simulink model "state_space_model_v0021"  (R2022b)
settings: Solver=VariableStepAuto  StartTime=0.0  StopTime=100  RelTol=1e-3
undefined symbols (not defined in the file): A_num, b_num, c, DiscIntNeverNeededParam, F_new, G, init_cond, Ts
libraries: simulink x1
settings Model: Creator=ninj2  LastModifiedBy=ninj2

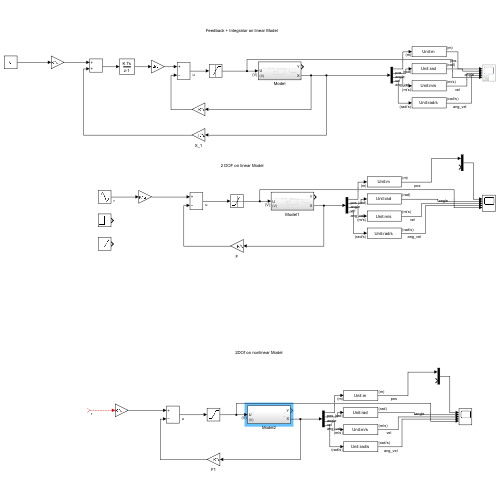
[thumbnail: Simulink's stored preview of the top-level diagram]
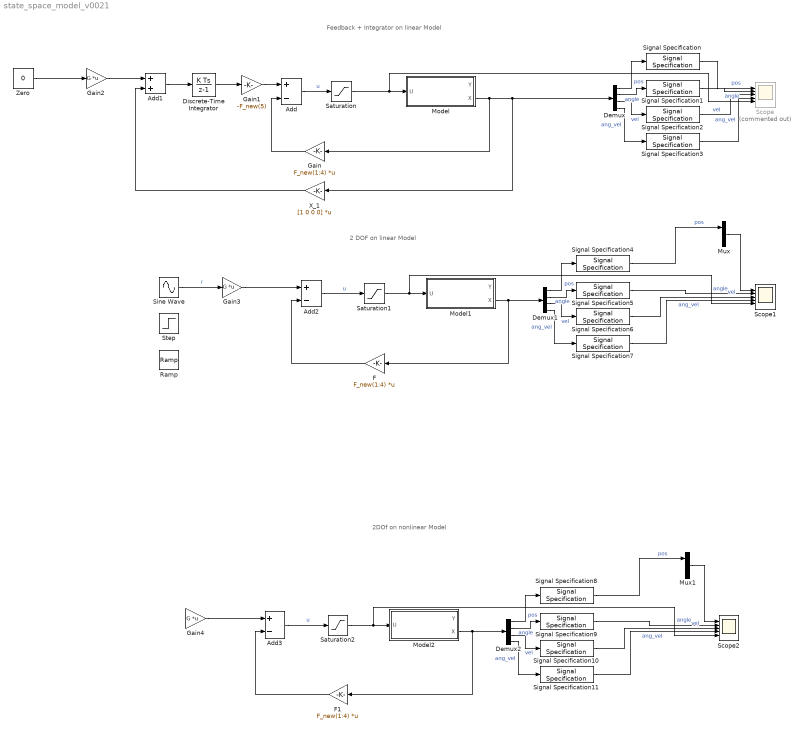
== system state_space_model_v0021 ==
  note: 2DOf on nonlinear Model
  note: 2 DOF on linear Model
  note: Feedback + Integrator on linear Model
  Add : Sum  Inputs=+-
  Add1 : Sum
  Add2 : Sum  Inputs=+-
  Add3 : Sum  Inputs=+-
  Demux : Demux
  Demux1 : Demux
  Demux2 : Demux
  Discrete-Time Integrator : DiscreteIntegrator  SampleTime=-1  ICPrevOutput=DiscIntNeverNeededParam  ICPrevScaledInput=DiscIntNeverNeededParam
  F : Gain  Gain=F_new(1:4)  Multiplication=Matrix(K*u)
  F1 : Gain  Gain=F_new(1:4)  Multiplication=Matrix(K*u)
  Gain : Gain  Gain=F_new(1:4)  Multiplication=Matrix(K*u)
  Gain1 : Gain  Gain=-F_new(5)
  Gain2 : Gain  Gain=G  Multiplication=Matrix(K*u)
  Gain3 : Gain  Gain=G  Multiplication=Matrix(K*u)
  Gain4 : Gain  Gain=G  Multiplication=Matrix(K*u)
  Model : Subsystem
  Model1 : Subsystem
  Model2 : Subsystem
  Mux : Mux  Inputs=2
  Mux1 : Mux  Inputs=2
  Ramp : simulink/Sources/Ramp  slope=0.01  start=0  InitialOutput=0
  Saturation : Saturate  UpperLimit=9  LowerLimit=-9
  Saturation1 : Saturate  UpperLimit=9  LowerLimit=-9
  Saturation2 : Saturate  UpperLimit=9  LowerLimit=-9
  Scope : Scope  Commented=on  NumInputPorts=5
  Scope1 : Scope  NumInputPorts=5
  Scope2 : Scope  NumInputPorts=5
  Signal Specification : SignalSpecification  Unit=m
  Signal Specification1 : SignalSpecification  Unit=rad
  Signal Specification10 : SignalSpecification  Unit=m/s
  Signal Specification11 : SignalSpecification  Unit=rad/s
  Signal Specification2 : SignalSpecification  Unit=m/s
  Signal Specification3 : SignalSpecification  Unit=rad/s
  Signal Specification4 : SignalSpecification  Unit=m
  Signal Specification5 : SignalSpecification  Unit=rad
  Signal Specification6 : SignalSpecification  Unit=m/s
  Signal Specification7 : SignalSpecification  Unit=rad/s
  Signal Specification8 : SignalSpecification  Unit=m
  Signal Specification9 : SignalSpecification  Unit=rad
  Sine Wave : Sin  Amplitude=0.05  Frequency=0.3  SampleTime=0
  Step : Step  After=0.05  SampleTime=0
  X_1 : Gain  Gain=[1 0 0 0]  Multiplication=Matrix(K*u)
  Zero : Constant  Value=0  OutDataTypeStr=Inherit: Inherit via back propagation
  wires:
  Add/1 -> Saturation/1  "u"
  Model/2(X) -> Gain/1, X_1/1, Demux/1
  Gain/1 -> Add/2
  Zero/1 -> Gain2/1
  Add1/1 -> Discrete-Time Integrator/1
  Discrete-Time Integrator/1 -> Gain1/1
  X_1/1 -> Add1/2
  Gain1/1 -> Add/1
  Demux/1 -> Signal Specification/1  "pos"
  Demux/2 -> Signal Specification1/1  "angle"
  Demux/3 -> Signal Specification2/1  "vel"
  Demux/4 -> Signal Specification3/1  "ang_vel"
  Signal Specification/1 -> Scope/1  "pos"
  Signal Specification1/1 -> Scope/2  "angle"
  Signal Specification2/1 -> Scope/3  "vel"
  Signal Specification3/1 -> Scope/4  "ang_vel"
  Saturation/1 -> Scope/5, Model/1(U)
  Saturation1/1 -> Scope1/5, Model1/1(U)
  Add2/1 -> Saturation1/1  "u"
  Demux1/1 -> Signal Specification4/1  "pos"
  Signal Specification7/1 -> Scope1/4  "ang_vel"
  Signal Specification6/1 -> Scope1/3  "vel"
  F/1 -> Add2/2
  Demux1/3 -> Signal Specification6/1  "vel"
  Signal Specification4/1 -> Mux/1  "pos"
  Demux1/4 -> Signal Specification7/1  "ang_vel"
  Signal Specification5/1 -> Scope1/2  "angle"
  Model1/2(X) -> F/1, Demux1/1
  Demux1/2 -> Signal Specification5/1  "angle"
  Gain3/1 -> Add2/1
  Mux/1 -> Scope1/1
  Gain2/1 -> Add1/1
  Sine Wave/1 -> Gain3/1  "r"
  Demux2/3 -> Signal Specification10/1  "vel"
  Signal Specification9/1 -> Scope2/2  "angle"
  Mux1/1 -> Scope2/1
  Demux2/4 -> Signal Specification11/1  "ang_vel"
  Gain4/1 -> Add3/1
  Signal Specification11/1 -> Scope2/4  "ang_vel"
  Demux2/2 -> Signal Specification9/1  "angle"
  Model2/2(X) -> F1/1, Demux2/1
  ? -> Gain4/1  "r"
  Saturation2/1 -> Scope2/5, Model2/1(U)
  Signal Specification8/1 -> Mux1/1  "pos"
  Demux2/1 -> Signal Specification8/1  "pos"
  F1/1 -> Add3/2
  Signal Specification10/1 -> Scope2/3  "vel"
  Add3/1 -> Saturation2/1  "u"

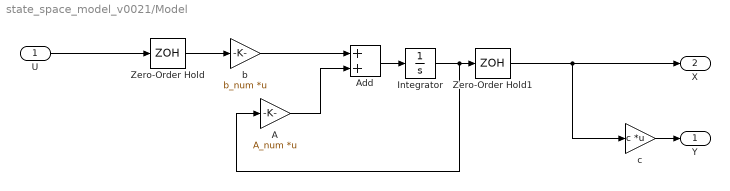
== system state_space_model_v0021/Model ==
  U : Inport  Unit=V
  A : Gain  Gain=A_num  Multiplication=Matrix(K*u)
  Add : Sum
  Integrator : Integrator  InitialCondition=init_cond
  Zero-Order Hold : ZeroOrderHold  SampleTime=Ts
  Zero-Order Hold1 : ZeroOrderHold  SampleTime=Ts
  b : Gain  Gain=b_num  Multiplication=Matrix(K*u)
  c : Gain  Gain=c  Multiplication=Matrix(K*u)
  Y : Outport
  X : Outport  Port=2
  wires:
  A/1 -> Add/2
  Add/1 -> Integrator/1
  Integrator/1 -> A/1, Zero-Order Hold1/1
  c/1 -> Y/1
  Zero-Order Hold/1 -> b/1
  b/1 -> Add/1
  Zero-Order Hold1/1 -> c/1, X/1
  U/1 -> Zero-Order Hold/1

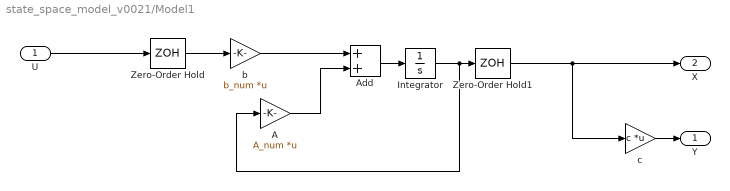
== system state_space_model_v0021/Model1 ==
  U : Inport  Unit=V
  A : Gain  Gain=A_num  Multiplication=Matrix(K*u)
  Add : Sum
  Integrator : Integrator  InitialCondition=init_cond
  Zero-Order Hold : ZeroOrderHold  SampleTime=Ts
  Zero-Order Hold1 : ZeroOrderHold  SampleTime=Ts
  b : Gain  Gain=b_num  Multiplication=Matrix(K*u)
  c : Gain  Gain=c  Multiplication=Matrix(K*u)
  Y : Outport
  X : Outport  Port=2
  wires:
  A/1 -> Add/2
  Add/1 -> Integrator/1
  Integrator/1 -> A/1, Zero-Order Hold1/1
  c/1 -> Y/1
  Zero-Order Hold/1 -> b/1
  b/1 -> Add/1
  Zero-Order Hold1/1 -> c/1, X/1
  U/1 -> Zero-Order Hold/1

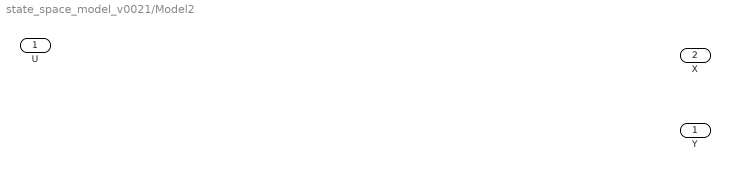
== system state_space_model_v0021/Model2 ==
  U : Inport  Unit=V
  Y : Outport
  X : Outport  Port=2
  wires:
  ? -> Y/1
